simulink model "ABMS_FK_Optimization"  (R2024a)
settings: Solver=ode45  StartTime=0.0  StopTime=t1(end)  MaxStep=1e-4  RelTol=1e-3
model workspace (MAT data in the model file):
  SDO_OutputTimes = 0
values from neighbouring files (symbols this model uses):
  c_floor = 62.8188429312    [ForwardKinematicsReadyOptimization.mat]
  cAnkle = 1000    [ForwardKinematicsReadyOptimization.mat]
  cHat = 1000    [ForwardKinematicsReadyOptimization.mat]
  cHip = 1000    [ForwardKinematicsReadyOptimization.mat]
  cKnee = 1000    [ForwardKinematicsReadyOptimization.mat]
  d = 0.005    [ForwardKinematicsReadyOptimization.mat]
  dt = 0.00194789579158    [ForwardKinematicsReadyOptimization.mat]
  footCoG_x = 0.048032    [ForwardKinematicsReadyOptimization.mat]
  footCoG_y = 0.03081    [ForwardKinematicsReadyOptimization.mat]
  footHeight = 0.06162    [ForwardKinematicsReadyOptimization.mat]
  footInertia = 0.00070433888961    [ForwardKinematicsReadyOptimization.mat]
  footLength = 0.24016    [ForwardKinematicsReadyOptimization.mat]
  footMass = 0.82215    [ForwardKinematicsReadyOptimization.mat]
  hatCoG = -0.05733504    [ForwardKinematicsReadyOptimization.mat]
  hatInertia = 1.9582821044    [ForwardKinematicsReadyOptimization.mat]
  k_floor = 2646.94405241    [ForwardKinematicsReadyOptimization.mat]
  kAnkle = 11643.6295541    [ForwardKinematicsReadyOptimization.mat]
  kHat = 20655.7189422    [ForwardKinematicsReadyOptimization.mat]
  kHip = 10850.9172876    [ForwardKinematicsReadyOptimization.mat]
  kKnee = 36599.3663246    [ForwardKinematicsReadyOptimization.mat]
  L = 1.58    [ForwardKinematicsReadyOptimization.mat]
  M = 56.7    [ForwardKinematicsReadyOptimization.mat]
  omega_ankle_L = [-1.72946807619 -1.75737353503 -1.78034856033 -1.79855294145 -1.81216431593 -1.82137637434 -1.82639701034 -1.82744643093 -1.82475524177 -1.81856252257 -1.80911390714 -1.79665968238 ... (500 elements, 500x1)]    [ForwardKinematicsReadyOptimization.mat]
  omega_ankle_R = [2.03625246317 1.87895799946 1.71908308042 1.55696000935 1.39292869416 1.22733586468 1.06053424947 0.892881711684 0.724740343936 0.556475522401 0.388454920876 0.221047485982 ... (500 elements, 500x1)]    [ForwardKinematicsReadyOptimization.mat]
  omega_hip_L = [-0.280611688679 -0.311570063188 -0.345107260568 -0.38110500203 -0.419429739456 -0.459933358207 -0.502453986364 -0.546816904373 -0.592835548257 -0.640312598834 -0.68904114874 -0.738805938443 ... (500 elements, 500x1)]    [ForwardKinematicsReadyOptimization.mat]
  omega_hip_R = [2.436874577 2.50137810017 2.56518693791 2.62820305906 2.690326825 2.7514571145 2.81149146904 2.87032625968 2.92785687598 2.98397793742 3.03858352766 3.09156745152 ... (500 elements, 500x1)]    [ForwardKinematicsReadyOptimization.mat]
  omega_knee_L = [1.96123814792 1.91418307718 1.85419760709 1.78297919547 1.70210911406 1.61305682274 1.51718435711 1.41575071667 1.30991624212 1.20074697044 1.08921895698 0.976222554764 ... (500 elements, 500x1)]    [ForwardKinematicsReadyOptimization.mat]
  omega_knee_R = [-6.31491022355 -6.2996719536 -6.27749939257 -6.24831489493 -6.21206519479 -6.168721658 -6.11828036625 -6.06076203398 -5.99621176048 -5.92469862101 -5.84631510196 -5.76117638659 ... (500 elements, 500x1)]    [ForwardKinematicsReadyOptimization.mat]
  shankCoG = 0.02604156    [ForwardKinematicsReadyOptimization.mat]
  shankInertia = 0.0363273974795    [ForwardKinematicsReadyOptimization.mat]
  shankLength = 0.38868    [ForwardKinematicsReadyOptimization.mat]
  shankMass = 2.63655    [ForwardKinematicsReadyOptimization.mat]
  theta_ankle_L = [0.104089190059 0.10089407725 0.0976495615316 0.094363371469 0.0910429873004 0.0876956182925 0.0843281827148 0.0809472904543 0.0775592282756 0.0741699477128 0.070785055563 0.0674098069326 ... (500 elements, 500x1)]    [ForwardKinematicsReadyOptimization.mat]
  theta_ankle_R = [0.268664443161 0.271247145186 0.273677847781 0.275939163558 0.27801459569 0.279888613303 0.281546720628 0.282975519613 0.284162765692 0.28509741648 0.285769673205 0.286171014728 ... (500 elements, 500x1)]    [ForwardKinematicsReadyOptimization.mat]
  theta_hip_L = [0.203866490768 0.203326556251 0.202708469588 0.202008986109 0.201225063456 0.20035388195 0.199392863962 0.198339692183 0.197192326665 0.195949020524 0.194608334197 0.19316914817 ... (500 elements, 500x1)]    [ForwardKinematicsReadyOptimization.mat]
  theta_hip_R = [-0.0372016659367 -0.0333395086271 -0.0292594880672 -0.0249651189751 -0.0204604325022 -0.0157499604189 -0.0108387175733 -0.00573218271268 -0.000436277763004 0.00504265433304 0.010697873109 0.0165222652855 ... (500 elements, 500x1)]    [ForwardKinematicsReadyOptimization.mat]
  theta_knee_L = [-0.239993153363 -0.245883098322 -0.251093519717 -0.255698925452 -0.259765380933 -0.263351270801 -0.266508012215 -0.269280721542 -0.271708836309 -0.273826694261 -0.275664071344 -0.277246680395 ... (500 elements, 500x1)]    [ForwardKinematicsReadyOptimization.mat]
  theta_knee_R = [-0.820430486691 -0.832341256015 -0.844266598336 -0.856189608949 -0.868093439005 -0.879961330014 -0.891776648203 -0.903522918602 -0.915183858758 -0.926743411958 -0.938185779838 -0.949495454282 ... (500 elements, 500x1)]    [ForwardKinematicsReadyOptimization.mat]
  thighCoG = 0.0259357    [ForwardKinematicsReadyOptimization.mat]
  thighInertia = 0.0886409590374    [ForwardKinematicsReadyOptimization.mat]
  thighLength = 0.3871    [ForwardKinematicsReadyOptimization.mat]
  thighMass = 5.67    [ForwardKinematicsReadyOptimization.mat]
  x_hip = [-8.44173174878e-05 0.00319684354612 0.00644879199438 0.00967154739147 0.0128652983927 0.0160302986852 0.0191668628036 0.0222753620261 0.0253562203613 0.0284099106285 0.0314369506394 0.0344378994863 ... (500 elements, 500x1)]    [ForwardKinematicsReadyOptimization.mat]
  y_hip = [0.786844713626 0.786912596344 0.786989490296 0.787076184105 0.787173456036 0.787282069444 0.787402768296 0.787536272813 0.787683275238 0.787844435773 0.788020378698 0.788211688702 ... (500 elements, 500x1)]    [ForwardKinematicsReadyOptimization.mat]
undefined symbols (not defined in the file or in its folder): omega_hat, X, Y, y_heel, Z
libraries: nesl_utility x77, sm_lib x60
(part 2 of 3)

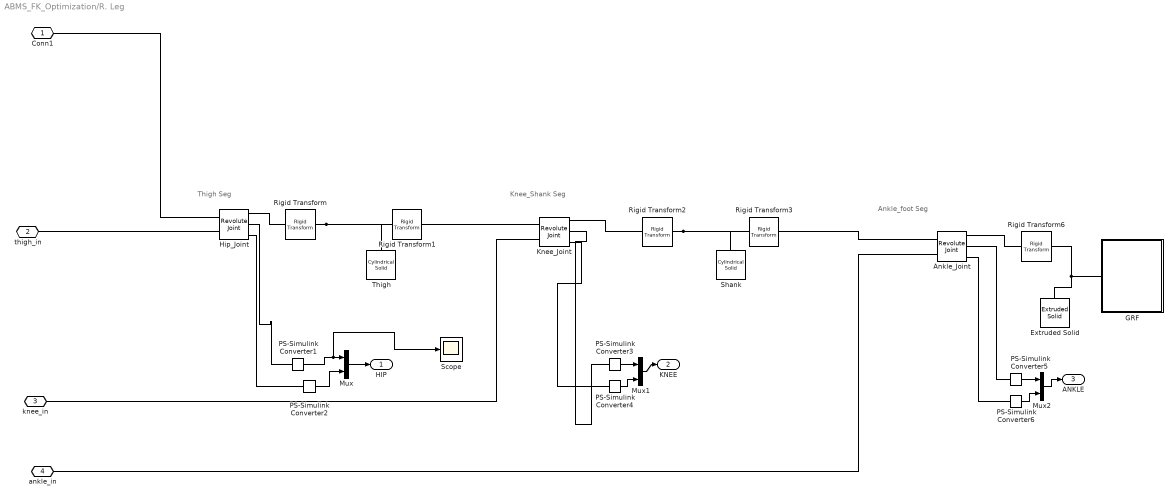
== system ABMS_FK_Optimization/R. Leg ==
  note: Ankle_foot Seg
  note: Knee_Shank Seg
  note: Thigh Seg
  Ankle_Joint : sm_lib/Joints/Revolute Joint  JointMode=Normal  CompositeWrenchDir=FollowerOnBase  CompositeWrenchFrame=BaseFrame  SenseConstraintForce=off  SenseConstraintTorque=off  SenseTotalForce=off  SenseTotalTorque=off  PositionTargetSpecify=on  PositionTargetPriority=High  PositionTargetValue=theta_ankle_R(1)  PositionTargetValueUnits=rad  VelocityTargetSpecify=on  VelocityTargetPriority=High  VelocityTargetValue=omega_ankle_R(1)  VelocityTargetValueUnits=rad/s  EquilibriumPosition=0  EquilibriumPositionUnits=deg  SpringStiffness=0  SpringStiffnessUnits=N*m/deg  DampingCoefficient=0  DampingCoefficientUnits=N*m/(deg/s)  LowerLimitSpecify=off  LowerLimitBound=-90  LowerLimitBoundUnits=deg  LowerLimitStiffness=1e4  LowerLimitStiffnessUnits=N*m/deg  LowerLimitDamping=10  LowerLimitDampingUnits=N*m/(deg/s)  LowerLimitTransitionRegionWidth=0.1  LowerLimitTransitionRegionWidthUnits=deg  UpperLimitSpecify=off  UpperLimitBound=90  UpperLimitBoundUnits=deg  UpperLimitStiffness=1e4  UpperLimitStiffnessUnits=N*m/deg  UpperLimitDamping=10  UpperLimitDampingUnits=N*m/(deg/s)  UpperLimitTransitionRegionWidth=0.1  UpperLimitTransitionRegionWidthUnits=deg  TorqueActuationMode=InputTorque  MotionActuationMode=ComputedMotion  SensePosition=on  SenseVelocity=on  SenseAcceleration=off  SenseTorqueForce=off  SenseLowerLimitTorqueForce=off  SenseUpperLimitTorqueForce=off
  Extruded Solid : sm_lib/Body Elements/Extruded Solid  ExtrusionType=General  PolygonNumSides=3  PolygonOuterRadius=footLength  PolygonOuterRadiusUnits=m  ExportEntireGeometry=off  ExtrusionCrossSection=[0 0; footLength 0; L*.0204 footHeight]  ExtrusionCrossSectionUnits=m  ExportConvexHullGeometry=off  ExtrusionLength=d  ExtrusionLengthUnits=m  InertiaType=Custom  BasedOnType=Mass  Density=1000  DensityUnits=kg/m^3  Mass=footMass  MassUnits=kg  CenterOfMass=[footCoG_x footCoG_y 0]  CenterOfMassUnits=m  MomentsOfInertia=[1 1 footInertia]  MomentsOfInertiaUnits=kg*m^2  ProductsOfInertia=[0 0 0]  ProductsOfInertiaUnits=kg*m^2  GraphicType=FromGeometry  MarkerShape=Sphere  MarkerSize=10  GraphicVisPropType=SimpleVisualProperties  GraphicDiffuseColor=[1.0 0.0 0.2]  GraphicOpacity=1.0  GraphicSpecularColor=[0.5 0.5 0.5 1.0]  GraphicAmbientColor=[0.15 0.15 0.15 1.0]  GraphicEmissiveColor=[0.0 0.0 0.0 1.0]  GraphicShininess=75  DoExposeReferenceFrame=on  SerializedFrames=<Frames><Frame><Id>Frame1</Id><Value><Name>CG</Name><Origin><Source>CenterOfMassFrame</Source><FeatureName></FeatureName></Origin><PrimaryAxis><DefinedDirection>+Z</DefinedDirection><Source>ReferenceFrame</Source><SourceDirection>+Z</SourceDirection><FeatureName></FeatureName></PrimaryAxis><SecondaryAxis><DefinedDirection>+X</DefinedDirection><Source>ReferenceFrame</Source><SourceDirection>+X</SourceDirection><FeatureName></FeatureName></SecondaryAxis></Value></Frame></Frames>
  GRF : Subsystem
  Hip_Joint : sm_lib/Joints/Revolute Joint  JointMode=Normal  CompositeWrenchDir=BaseOnFollower  CompositeWrenchFrame=BaseFrame  SenseConstraintForce=off  SenseConstraintTorque=off  SenseTotalForce=off  SenseTotalTorque=off  PositionTargetSpecify=on  PositionTargetPriority=High  PositionTargetValue=theta_hip_R(1)  PositionTargetValueUnits=rad  VelocityTargetSpecify=on  VelocityTargetPriority=High  VelocityTargetValue=omega_hip_R(1)  VelocityTargetValueUnits=rad/s  EquilibriumPosition=0  EquilibriumPositionUnits=deg  SpringStiffness=0  SpringStiffnessUnits=N*m/deg  DampingCoefficient=0  DampingCoefficientUnits=N*m/(deg/s)  LowerLimitSpecify=off  LowerLimitBound=-90  LowerLimitBoundUnits=deg  LowerLimitStiffness=1e4  LowerLimitStiffnessUnits=N*m/deg  LowerLimitDamping=10  LowerLimitDampingUnits=N*m/(deg/s)  LowerLimitTransitionRegionWidth=0.1  LowerLimitTransitionRegionWidthUnits=deg  UpperLimitSpecify=off  UpperLimitBound=90  UpperLimitBoundUnits=deg  UpperLimitStiffness=1e4  UpperLimitStiffnessUnits=N*m/deg  UpperLimitDamping=10  UpperLimitDampingUnits=N*m/(deg/s)  UpperLimitTransitionRegionWidth=0.1  UpperLimitTransitionRegionWidthUnits=deg  TorqueActuationMode=InputTorque  MotionActuationMode=ComputedMotion  SensePosition=on  SenseVelocity=on  SenseAcceleration=off  SenseTorqueForce=off  SenseLowerLimitTorqueForce=off  SenseUpperLimitTorqueForce=off
  Knee_Joint : sm_lib/Joints/Revolute Joint  JointMode=Normal  CompositeWrenchDir=FollowerOnBase  CompositeWrenchFrame=BaseFrame  SenseConstraintForce=off  SenseConstraintTorque=off  SenseTotalForce=off  SenseTotalTorque=off  PositionTargetSpecify=on  PositionTargetPriority=High  PositionTargetValue=theta_knee_R(1)  PositionTargetValueUnits=rad  VelocityTargetSpecify=on  VelocityTargetPriority=High  VelocityTargetValue=omega_knee_R(1)  VelocityTargetValueUnits=rad/s  EquilibriumPosition=0  EquilibriumPositionUnits=deg  SpringStiffness=0  SpringStiffnessUnits=N*m/deg  DampingCoefficient=0  DampingCoefficientUnits=N*m/(deg/s)  LowerLimitSpecify=off  LowerLimitBound=-90  LowerLimitBoundUnits=deg  LowerLimitStiffness=1e4  LowerLimitStiffnessUnits=N*m/deg  LowerLimitDamping=10  LowerLimitDampingUnits=N*m/(deg/s)  LowerLimitTransitionRegionWidth=0.1  LowerLimitTransitionRegionWidthUnits=deg  UpperLimitSpecify=off  UpperLimitBound=90  UpperLimitBoundUnits=deg  UpperLimitStiffness=1e4  UpperLimitStiffnessUnits=N*m/deg  UpperLimitDamping=10  UpperLimitDampingUnits=N*m/(deg/s)  UpperLimitTransitionRegionWidth=0.1  UpperLimitTransitionRegionWidthUnits=deg  TorqueActuationMode=InputTorque  MotionActuationMode=ComputedMotion  SensePosition=on  SenseVelocity=on  SenseAcceleration=off  SenseTorqueForce=off  SenseLowerLimitTorqueForce=off  SenseUpperLimitTorqueForce=off
  Mux : Mux  Inputs=2
  Mux1 : Mux  Inputs=2
  Mux2 : Mux  Inputs=2
  PS-Simulink Converter{1..6} (6 alike) : nesl_utility/PS-Simulink Converter  PhysicalDomain=network_engine_domain  SubClassName=ps_output  LeftPortType=input  RightPortType=output  PseudoPeriodic=off  Frequencies=[]  VectorFormat=1-D array  Unit=inherit  AffineConversion=off
  Rigid Transform : sm_lib/Frames and Transforms/Rigid Transform  RotationMethod=StandardAxis  FollAlignAxisA=+X  BaseAlignAxisA=+Y  FollAlignAxisB=+Y  BaseAlignAxisB=+Z  RotationStandardAxis=+X  RotationAngle=90  RotationAngleUnits=deg  RotationArbitraryAxis=[0 0 1]  RotationSequenceAxes=FollowerAxes  RotationSequence=XYX  RotationSequenceAngles=[0 0 0]  RotationSequenceAnglesUnits=deg  RotationMatrix=[1 0 0; 0 1 0; 0 0 1]  Quaternion=[1 0 0 0]  TranslationMethod=Cartesian  TranslationCartesianOffset=[0 0 thighLength/2]  TranslationCartesianOffsetUnits=m  TranslationStandardAxis=+Z  TranslationStandardOffset=thighLength/2  TranslationStandardOffsetUnits=m  TranslationROffset=0  TranslationROffsetUnits=m  TranslationThetaOffset=0  TranslationThetaOffsetUnits=deg  TranslationZOffset=0  TranslationZOffsetUnits=m
  Rigid Transform1 : sm_lib/Frames and Transforms/Rigid Transform  RotationMethod=StandardAxis  FollAlignAxisA=+X  BaseAlignAxisA=+Y  FollAlignAxisB=+Y  BaseAlignAxisB=+Z  RotationStandardAxis=+X  RotationAngle=90  RotationAngleUnits=deg  RotationArbitraryAxis=[0 0 1]  RotationSequenceAxes=FollowerAxes  RotationSequence=XYX  RotationSequenceAngles=[0 0 0]  RotationSequenceAnglesUnits=deg  RotationMatrix=[1 0 0; 0 1 0; 0 0 1]  Quaternion=[1 0 0 0]  TranslationMethod=StandardAxis  TranslationCartesianOffset=[0 0 0]  TranslationCartesianOffsetUnits=m  TranslationStandardAxis=-Z  TranslationStandardOffset=thighLength/2  TranslationStandardOffsetUnits=m  TranslationROffset=0  TranslationROffsetUnits=m  TranslationThetaOffset=0  TranslationThetaOffsetUnits=deg  TranslationZOffset=0  TranslationZOffsetUnits=m
  Rigid Transform2 : sm_lib/Frames and Transforms/Rigid Transform  RotationMethod=StandardAxis  FollAlignAxisA=+X  BaseAlignAxisA=+Y  FollAlignAxisB=+Y  BaseAlignAxisB=+Z  RotationStandardAxis=+X  RotationAngle=90  RotationAngleUnits=deg  RotationArbitraryAxis=[0 0 1]  RotationSequenceAxes=FollowerAxes  RotationSequence=XYX  RotationSequenceAngles=[0 0 0]  RotationSequenceAnglesUnits=deg  RotationMatrix=[1 0 0; 0 1 0; 0 0 1]  Quaternion=[1 0 0 0]  TranslationMethod=StandardAxis  TranslationCartesianOffset=[0 0 0]  TranslationCartesianOffsetUnits=m  TranslationStandardAxis=+Z  TranslationStandardOffset=shankLength/2  TranslationStandardOffsetUnits=m  TranslationROffset=0  TranslationROffsetUnits=m  TranslationThetaOffset=0  TranslationThetaOffsetUnits=deg  TranslationZOffset=0  TranslationZOffsetUnits=m
  Rigid Transform3 : sm_lib/Frames and Transforms/Rigid Transform  RotationMethod=StandardAxis  FollAlignAxisA=+X  BaseAlignAxisA=+Y  FollAlignAxisB=+Y  BaseAlignAxisB=+Z  RotationStandardAxis=+X  RotationAngle=90  RotationAngleUnits=deg  RotationArbitraryAxis=[0 0 1]  RotationSequenceAxes=FollowerAxes  RotationSequence=XYX  RotationSequenceAngles=[0 0 0]  RotationSequenceAnglesUnits=deg  RotationMatrix=[1 0 0; 0 1 0; 0 0 1]  Quaternion=[1 0 0 0]  TranslationMethod=StandardAxis  TranslationCartesianOffset=[0 0 0]  TranslationCartesianOffsetUnits=m  TranslationStandardAxis=-Z  TranslationStandardOffset=shankLength/2  TranslationStandardOffsetUnits=m  TranslationROffset=0  TranslationROffsetUnits=m  TranslationThetaOffset=0  TranslationThetaOffsetUnits=deg  TranslationZOffset=0  TranslationZOffsetUnits=m
  Rigid Transform6 : sm_lib/Frames and Transforms/Rigid Transform  RotationMethod=None  FollAlignAxisA=+X  BaseAlignAxisA=+Y  FollAlignAxisB=+Y  BaseAlignAxisB=+Z  RotationStandardAxis=+Z  RotationAngle=0.0  RotationAngleUnits=deg  RotationArbitraryAxis=[0 0 1]  RotationSequenceAxes=FollowerAxes  RotationSequence=XYX  RotationSequenceAngles=[0 0 0]  RotationSequenceAnglesUnits=deg  RotationMatrix=[1 0 0; 0 1 0; 0 0 1]  Quaternion=[1 0 0 0]  TranslationMethod=Cartesian  TranslationCartesianOffset=[0.0204*L 0.039*L 0]  TranslationCartesianOffsetUnits=m  TranslationStandardAxis=+Z  TranslationStandardOffset=0  TranslationStandardOffsetUnits=m  TranslationROffset=0  TranslationROffsetUnits=m  TranslationThetaOffset=0  TranslationThetaOffsetUnits=deg  TranslationZOffset=0  TranslationZOffsetUnits=m
  Scope : Scope
  Shank : sm_lib/Body Elements/Cylindrical Solid  CylinderRadius=d/2  CylinderRadiusUnits=m  CylinderLength=shankLength  CylinderLengthUnits=m  ExportEntireGeometry=off  InertiaType=Custom  BasedOnType=Mass  Density=1000  DensityUnits=kg/m^3  Mass=shankMass  MassUnits=kg  CenterOfMass=[0 0 shankCoG]  CenterOfMassUnits=m  MomentsOfInertia=[shankInertia shankInertia 0]  MomentsOfInertiaUnits=kg*m^2  ProductsOfInertia=[0 0 0]  ProductsOfInertiaUnits=kg*m^2  GraphicType=FromGeometry  MarkerShape=Sphere  MarkerSize=10  GraphicVisPropType=SimpleVisualProperties  GraphicDiffuseColor=[0.0 0.2 1.0]  GraphicOpacity=1.0  GraphicSpecularColor=[0.5 0.5 0.5 1.0]  GraphicAmbientColor=[0.15 0.15 0.15 1.0]  GraphicEmissiveColor=[0.0 0.0 0.0 1.0]  GraphicShininess=75  DoExposeReferenceFrame=on  SerializedFrames=<Frames><Frame><Id>Frame1</Id><Value><Name>CG</Name><Origin><Source>CenterOfMassFrame</Source><FeatureName></FeatureName></Origin><PrimaryAxis><DefinedDirection>+Z</DefinedDirection><Source>ReferenceFrame</Source><SourceDirection>+Z</SourceDirection><FeatureName></FeatureName></PrimaryAxis><SecondaryAxis><DefinedDirection>+X</DefinedDirection><Source>ReferenceFrame</Source><SourceDirection>+X</SourceDirection><FeatureName></FeatureName></SecondaryAxis></Value></Frame></Frames>
  Thigh : sm_lib/Body Elements/Cylindrical Solid  CylinderRadius=d/2  CylinderRadiusUnits=m  CylinderLength=thighLength  CylinderLengthUnits=m  ExportEntireGeometry=off  InertiaType=Custom  BasedOnType=Mass  Density=1000  DensityUnits=kg/m^3  Mass=thighMass  MassUnits=kg  CenterOfMass=[0 0 thighCoG]  CenterOfMassUnits=m  MomentsOfInertia=[thighInertia thighInertia 0]  MomentsOfInertiaUnits=kg*m^2  ProductsOfInertia=[0 0 0]  ProductsOfInertiaUnits=kg*m^2  GraphicType=FromGeometry  MarkerShape=Sphere  MarkerSize=10  GraphicVisPropType=SimpleVisualProperties  GraphicDiffuseColor=[0.0 0.0 0.0]  GraphicOpacity=1.0  GraphicSpecularColor=[0.5 0.5 0.5 1.0]  GraphicAmbientColor=[0.15 0.15 0.15 1.0]  GraphicEmissiveColor=[0.0 0.0 0.0 1.0]  GraphicShininess=75  DoExposeReferenceFrame=on  SerializedFrames=<Frames><Frame><Id>Frame1</Id><Value><Name>CG</Name><Origin><Source>CenterOfMassFrame</Source><FeatureName></FeatureName></Origin><PrimaryAxis><DefinedDirection>+Z</DefinedDirection><Source>ReferenceFrame</Source><SourceDirection>+Z</SourceDirection><FeatureName></FeatureName></PrimaryAxis><SecondaryAxis><DefinedDirection>+X</DefinedDirection><Source>ReferenceFrame</Source><SourceDirection>+X</SourceDirection><FeatureName></FeatureName></SecondaryAxis></Value></Frame></Frames>
  Conn1 : PMIOPort  Side=Left
  thigh_in : PMIOPort  Port=2  Side=Left
  knee_in : PMIOPort  Port=3  Side=Left
  ankle_in : PMIOPort  Port=4  Side=Left
  HIP : Outport
  KNEE : Outport  Port=2
  ANKLE : Outport  Port=3
  wires:
  PS-Simulink Converter2/1 -> Mux/2
  PS-Simulink Converter4/1 -> Mux1/2
  PS-Simulink Converter1/1 -> Scope/1, Mux/1
  Mux/1 -> HIP/1
  PS-Simulink Converter3/1 -> Mux1/1
  Mux1/1 -> KNEE/1
  PS-Simulink Converter5/1 -> Mux2/1
  Mux2/1 -> ANKLE/1
  PS-Simulink Converter6/1 -> Mux2/2
  connections:
  Rigid Transform/LConn1 -- Rigid Transform1/LConn1 -- Thigh/RConn1
  Knee_Joint/LConn1 -- Rigid Transform1/RConn1
  Hip_Joint/RConn1 -- Rigid Transform/RConn1
  Rigid Transform2/LConn1 -- Shank/RConn1 -- Rigid Transform3/LConn1
  Rigid Transform6/RConn1 -- Ankle_Joint/RConn1
  Rigid Transform2/RConn1 -- Knee_Joint/RConn1
  Rigid Transform3/RConn1 -- Ankle_Joint/LConn1
  Hip_Joint/LConn1 -- Conn1/RConn1
  PS-Simulink Converter1/LConn1 -- Hip_Joint/RConn2
  Extruded Solid/RConn1 -- GRF/LConn1 -- Rigid Transform6/LConn1
  PS-Simulink Converter4/LConn1 -- Knee_Joint/RConn3
  PS-Simulink Converter3/LConn1 -- Knee_Joint/RConn2
  PS-Simulink Converter2/LConn1 -- Hip_Joint/RConn3
  Ankle_Joint/RConn2 -- PS-Simulink Converter5/LConn1
  PS-Simulink Converter6/LConn1 -- Ankle_Joint/RConn3
  thigh_in/RConn1 -- Hip_Joint/LConn2
  knee_in/RConn1 -- Knee_Joint/LConn2
  ankle_in/RConn1 -- Ankle_Joint/LConn2

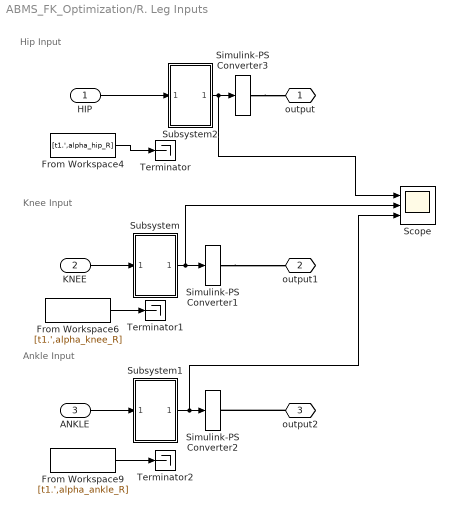
== system ABMS_FK_Optimization/R. Leg Inputs ==
  note: Ankle Input
  note: Knee Input
  note: Hip Input
  HIP : Inport
  KNEE : Inport  Port=2
  ANKLE : Inport  Port=3
  From Workspace4 : FromWorkspace  VariableName=[t1.',alpha_hip_R]  SampleTime=dt
  From Workspace6 : FromWorkspace  VariableName=[t1.',alpha_knee_R]  SampleTime=dt
  From Workspace9 : FromWorkspace  VariableName=[t1.',alpha_ankle_R]  SampleTime=dt
  Scope : Scope  NumInputPorts=3
  Simulink-PS Converter1 : nesl_utility/Simulink-PS Converter  PhysicalDomain=network_engine_domain  SubClassName=ps_input  LeftPortType=input  RightPortType=output  PseudoPeriodic=off  Frequencies=[]  NoiseDistribution=none  NoiseParameters=[]  Unit=1  AffineConversion=off  FilteringAndDerivatives=provide  SimscapeFilterOrder=2  InputFilterTimeConstant=0.001  UdotUserProvided=0
  Simulink-PS Converter2 : nesl_utility/Simulink-PS Converter  PhysicalDomain=network_engine_domain  SubClassName=ps_input  LeftPortType=input  RightPortType=output  PseudoPeriodic=off  Frequencies=[]  NoiseDistribution=none  NoiseParameters=[]  Unit=1  AffineConversion=off  FilteringAndDerivatives=provide  SimscapeFilterOrder=2  InputFilterTimeConstant=0.001  UdotUserProvided=0
  Simulink-PS Converter3 : nesl_utility/Simulink-PS Converter  PhysicalDomain=network_engine_domain  SubClassName=ps_input  LeftPortType=input  RightPortType=output  PseudoPeriodic=off  Frequencies=[]  NoiseDistribution=none  NoiseParameters=[]  Unit=1  AffineConversion=off  FilteringAndDerivatives=provide  SimscapeFilterOrder=2  InputFilterTimeConstant=0.001  UdotUserProvided=0
  Subsystem : Subsystem
  Subsystem1 : Subsystem
  Subsystem2 : Subsystem
  Terminator : Terminator
  Terminator1 : Terminator
  Terminator2 : Terminator
  output : PMIOPort  Side=Right
  output1 : PMIOPort  Port=2  Side=Right
  output2 : PMIOPort  Port=3  Side=Right
  wires:
  KNEE/1 -> Subsystem/1(In1)
  Subsystem/1(Out1) -> Scope/2, Simulink-PS Converter1/1
  ANKLE/1 -> Subsystem1/1(In1)
  Subsystem1/1(Out1) -> Scope/3, Simulink-PS Converter2/1
  HIP/1 -> Subsystem2/1(1)
  Subsystem2/1(Out1) -> Scope/1, Simulink-PS Converter3/1
  From Workspace4/1 -> Terminator/1
  From Workspace6/1 -> Terminator1/1
  From Workspace9/1 -> Terminator2/1
  connections:
  output2/RConn1 -- Simulink-PS Converter2/RConn1
  Simulink-PS Converter1/RConn1 -- output1/RConn1
  Simulink-PS Converter3/RConn1 -- output/RConn1

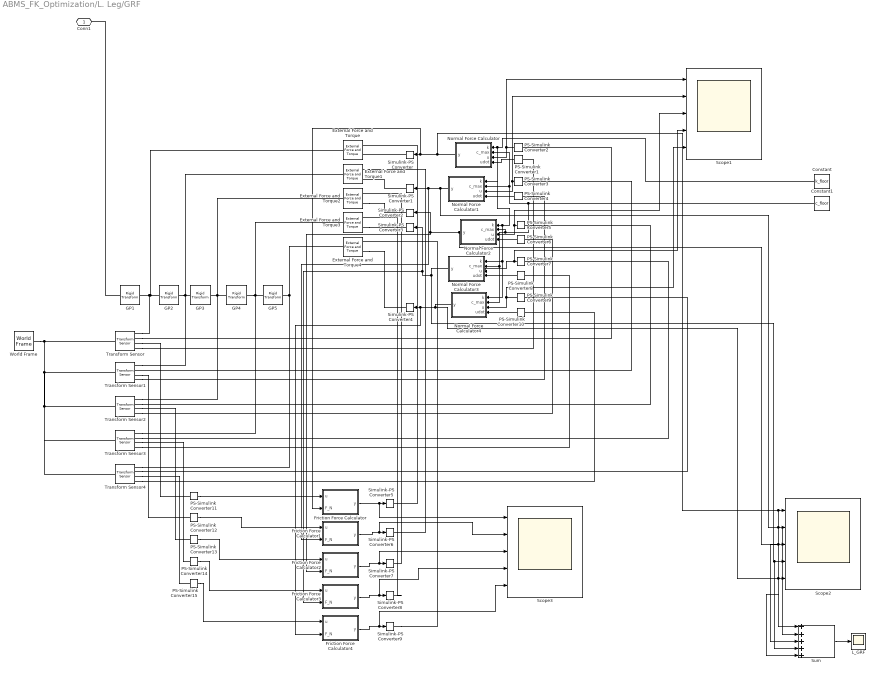
== system ABMS_FK_Optimization/L. Leg/GRF ==
  Constant : Constant  Value=k_floor
  Constant1 : Constant  Value=c_floor
  External Force and Torque{,1..4} (5 alike) : sm_lib/Forces and Torques/External Force and Torque  EnableForceX=on  EnableForceY=on  EnableForceZ=off  EnableForce=off  ForceResolutionFrame=World  EnableTorqueX=off  EnableTorqueY=off  EnableTorqueZ=off  EnableTorque=off  TorqueResolutionFrame=AttachedFrame
  Friction Force Calculator : MATLAB Function  TreatAsAtomicUnit=on
  Friction Force Calculator1 : MATLAB Function  TreatAsAtomicUnit=on
  Friction Force Calculator2 : MATLAB Function  TreatAsAtomicUnit=on
  Friction Force Calculator3 : MATLAB Function  TreatAsAtomicUnit=on
  Friction Force Calculator4 : MATLAB Function  TreatAsAtomicUnit=on
  GP1 : sm_lib/Frames and Transforms/Rigid Transform  RotationMethod=None  FollAlignAxisA=+X  BaseAlignAxisA=+Y  FollAlignAxisB=+Y  BaseAlignAxisB=+Z  RotationStandardAxis=+Z  RotationAngle=0.0  RotationAngleUnits=deg  RotationArbitraryAxis=[0 0 1]  RotationSequenceAxes=FollowerAxes  RotationSequence=XYX  RotationSequenceAngles=[0 0 0]  RotationSequenceAnglesUnits=deg  RotationMatrix=[1 0 0; 0 1 0; 0 0 1]  Quaternion=[1 0 0 0]  TranslationMethod=None  TranslationCartesianOffset=[0 0 0]  TranslationCartesianOffsetUnits=m  TranslationStandardAxis=-X  TranslationStandardOffset=d/2  TranslationStandardOffsetUnits=m  TranslationROffset=0  TranslationROffsetUnits=m  TranslationThetaOffset=0  TranslationThetaOffsetUnits=deg  TranslationZOffset=0  TranslationZOffsetUnits=m
  GP{2..5} (4 alike) : sm_lib/Frames and Transforms/Rigid Transform  RotationMethod=None  FollAlignAxisA=+X  BaseAlignAxisA=+Y  FollAlignAxisB=+Y  BaseAlignAxisB=+Z  RotationStandardAxis=+Z  RotationAngle=0.0  RotationAngleUnits=deg  RotationArbitraryAxis=[0 0 1]  RotationSequenceAxes=FollowerAxes  RotationSequence=XYX  RotationSequenceAngles=[0 0 0]  RotationSequenceAnglesUnits=deg  RotationMatrix=[1 0 0; 0 1 0; 0 0 1]  Quaternion=[1 0 0 0]  TranslationMethod=StandardAxis  TranslationCartesianOffset=[0 0 0]  TranslationCartesianOffsetUnits=m  TranslationStandardAxis=+X  TranslationStandardOffset=footLength/4  TranslationStandardOffsetUnits=m  TranslationROffset=0  TranslationROffsetUnits=m  TranslationThetaOffset=0  TranslationThetaOffsetUnits=deg  TranslationZOffset=0  TranslationZOffsetUnits=m
  L_GRF : Scope
  Normal Force Calculator : MATLAB Function  TreatAsAtomicUnit=on
  Normal Force Calculator1 : MATLAB Function  TreatAsAtomicUnit=on
  Normal Force Calculator2 : MATLAB Function  TreatAsAtomicUnit=on
  Normal Force Calculator3 : MATLAB Function  TreatAsAtomicUnit=on
  Normal Force Calculator4 : MATLAB Function  TreatAsAtomicUnit=on
  PS-Simulink Converter{1..15} (15 alike) : nesl_utility/PS-Simulink Converter  PhysicalDomain=network_engine_domain  SubClassName=ps_output  LeftPortType=input  RightPortType=output  PseudoPeriodic=off  Frequencies=[]  VectorFormat=1-D array  Unit=inherit  AffineConversion=off
  Scope1 : Scope  NumInputPorts=5
  Scope2 : Scope  NumInputPorts=5
  Scope3 : Scope  NumInputPorts=5
  Simulink-PS Converter{,1..9} (10 alike) : nesl_utility/Simulink-PS Converter  PhysicalDomain=network_engine_domain  SubClassName=ps_input  LeftPortType=input  RightPortType=output  PseudoPeriodic=off  Frequencies=[]  NoiseDistribution=none  NoiseParameters=[]  Unit=1  AffineConversion=off  FilteringAndDerivatives=provide  SimscapeFilterOrder=1  InputFilterTimeConstant=0.001  UdotUserProvided=0
  Sum : Sum  Inputs=+++++
  Transform Sensor{,1..4} (5 alike) : sm_lib/Frames and Transforms/Transform Sensor  MeasurementFrame=World  RotationSequence=XYX  SenseAngle=off  SenseAxis=off  SenseQ=off  SenseR=off  SenseRotationSequence=off  SenseOmegaX=off  SenseOmegaY=off  SenseOmegaZ=off  SenseOmega=off  SenseQDot=off  SenseRDot=off  SenseRotationSequenceDot=off  SenseAlphaX=off  SenseAlphaY=off  SenseAlphaZ=off  SenseAlpha=off  SenseQDDot=off  SenseRDDot=off  SenseX=off  SenseY=on  SenseZ=off  SenseXYZ=off  SenseRad=off  SenseAzim=off  SenseDist=off  SenseInc=off  SenseXDot=on  SenseYDot=on  SenseZDot=off  SenseXYZDot=off  SenseRadDot=off  SenseAzimDot=off  SenseDistDot=off  SenseIncDot=off  SenseXDDot=off  SenseYDDot=off  SenseZDDot=off  SenseXYZDDot=off  SenseRadDDot=off  SenseAzimDDot=off  SenseDistDDot=off  SenseIncDDot=off
  World Frame : sm_lib/Frames and Transforms/World Frame
  Conn1 : PMIOPort  Side=Left
  wires:
  PS-Simulink Converter2/1 -> Scope1/1, Normal Force Calculator/3(u)
  Normal Force Calculator4/1(y) -> Sum/5, Scope2/5, Friction Force Calculator4/2(F_N), Simulink-PS Converter4/1
  Friction Force Calculator3/1(y) -> Scope3/4, Simulink-PS Converter8/1
  Normal Force Calculator/1(y) -> Sum/1, Scope2/1, Friction Force Calculator/2(F_N), Simulink-PS Converter/1
  PS-Simulink Converter9/1 -> Normal Force Calculator4/3(u), Scope1/5
  Friction Force Calculator4/1(y) -> Scope3/5, Simulink-PS Converter9/1
  PS-Simulink Converter5/1 -> Normal Force Calculator2/3(u), Scope1/3
  PS-Simulink Converter15/1 -> Friction Force Calculator4/1(u)
  PS-Simulink Converter10/1 -> Normal Force Calculator4/4(udot)
  PS-Simulink Converter8/1 -> Normal Force Calculator3/4(udot)
  PS-Simulink Converter12/1 -> Friction Force Calculator1/1(u)
  Normal Force Calculator1/1(y) -> Sum/2, Scope2/2, Friction Force Calculator1/2(F_N), Simulink-PS Converter1/1
  PS-Simulink Converter13/1 -> Friction Force Calculator2/1(u)
  PS-Simulink Converter3/1 -> Normal Force Calculator1/3(u), Scope1/2
  PS-Simulink Converter4/1 -> Normal Force Calculator1/4(udot)
  Friction Force Calculator2/1(y) -> Scope3/3, Simulink-PS Converter7/1
  PS-Simulink Converter1/1 -> Normal Force Calculator/4(udot)
  Friction Force Calculator/1(y) -> Scope3/1, Simulink-PS Converter5/1
  Normal Force Calculator3/1(y) -> Scope2/4, Sum/4, Friction Force Calculator3/2(F_N), Simulink-PS Converter3/1
  PS-Simulink Converter7/1 -> Normal Force Calculator3/3(u), Scope1/4
  Constant1/1 -> Normal Force Calculator4/2(c_max), Normal Force Calculator3/2(c_max), Normal Force Calculator2/2(c_max), Normal Force Calculator1/2(c_max), Normal Force Calculator/2(c_max)
  PS-Simulink Converter6/1 -> Normal Force Calculator2/4(udot)
  Normal Force Calculator2/1(y) -> Sum/3, Scope2/3, Friction Force Calculator2/2(F_N), Simulink-PS Converter2/1
  Friction Force Calculator1/1(y) -> Scope3/2, Simulink-PS Converter6/1
  Sum/1 -> L_GRF/1
  Constant/1 -> Normal Force Calculator3/1(k), Normal Force Calculator4/1(k), Normal Force Calculator2/1(k), Normal Force Calculator1/1(k), Normal Force Calculator/1(k)
  PS-Simulink Converter14/1 -> Friction Force Calculator3/1(u)
  PS-Simulink Converter11/1 -> Friction Force Calculator/1(u)
  connections:
  Simulink-PS Converter5/RConn1 -- External Force and Torque/LConn1
  External Force and Torque2/LConn2 -- Simulink-PS Converter2/RConn1
  GP3/RConn1 -- External Force and Torque2/RConn1 -- Transform Sensor2/RConn1 -- GP4/LConn1
  GP2/LConn1 -- External Force and Torque/RConn1 -- Transform Sensor/RConn1 -- GP1/RConn1
  Transform Sensor2/RConn4 -- PS-Simulink Converter6/LConn1
  World Frame/RConn1 -- Transform Sensor4/LConn1 -- Transform Sensor3/LConn1 -- Transform Sensor2/LConn1 -- Transform Sensor1/LConn1 -- Transform Sensor/LConn1
  Transform Sensor3/RConn4 -- PS-Simulink Converter8/LConn1
  External Force and Torque1/LConn1 -- Simulink-PS Converter6/RConn1
  Transform Sensor3/RConn3 -- PS-Simulink Converter14/LConn1
  Transform Sensor4/RConn1 -- External Force and Torque4/RConn1 -- GP5/RConn1
  External Force and Torque3/LConn2 -- Simulink-PS Converter3/RConn1
  GP4/RConn1 -- External Force and Torque3/RConn1 -- Transform Sensor3/RConn1 -- GP5/LConn1
  Transform Sensor/RConn2 -- PS-Simulink Converter2/LConn1
  Transform Sensor2/RConn3 -- PS-Simulink Converter13/LConn1
  GP3/LConn1 -- External Force and Torque1/RConn1 -- Transform Sensor1/RConn1 -- GP2/RConn1
  Simulink-PS Converter7/RConn1 -- External Force and Torque2/LConn1
  Simulink-PS Converter8/RConn1 -- External Force and Torque3/LConn1
  PS-Simulink Converter3/LConn1 -- Transform Sensor1/RConn2
  Simulink-PS Converter1/RConn1 -- External Force and Torque1/LConn2
  Transform Sensor/RConn4 -- PS-Simulink Converter1/LConn1
  Transform Sensor4/RConn4 -- PS-Simulink Converter10/LConn1
  Transform Sensor4/RConn2 -- PS-Simulink Converter9/LConn1
  Transform Sensor/RConn3 -- PS-Simulink Converter11/LConn1
  Transform Sensor1/RConn4 -- PS-Simulink Converter4/LConn1
  Simulink-PS Converter/RConn1 -- External Force and Torque/LConn2
  Transform Sensor3/RConn2 -- PS-Simulink Converter7/LConn1
  Transform Sensor2/RConn2 -- PS-Simulink Converter5/LConn1
  Simulink-PS Converter9/RConn1 -- External Force and Torque4/LConn1
  Transform Sensor1/RConn3 -- PS-Simulink Converter12/LConn1
  Transform Sensor4/RConn3 -- PS-Simulink Converter15/LConn1
  External Force and Torque4/LConn2 -- Simulink-PS Converter4/RConn1
  GP1/LConn1 -- Conn1/RConn1

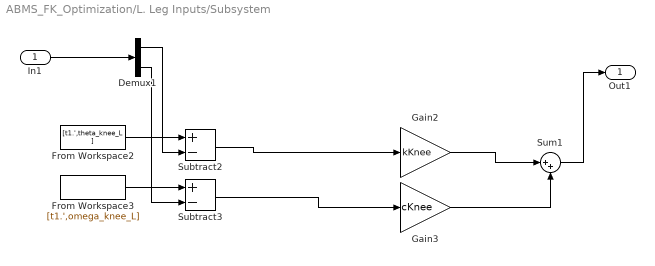
== system ABMS_FK_Optimization/L. Leg Inputs/Subsystem ==
  In1 : Inport
  Demux1 : Demux  Outputs=2
  From Workspace2 : FromWorkspace  VariableName=[t1.',theta_knee_L ]  SampleTime=dt
  From Workspace3 : FromWorkspace  VariableName=[t1.',omega_knee_L]  SampleTime=dt
  Gain2 : Gain  Gain=kKnee
  Gain3 : Gain  Gain=cKnee
  Subtract2 : Sum  Inputs=+-
  Subtract3 : Sum  Inputs=+-
  Sum1 : Sum  Inputs=|++
  Out1 : Outport
  wires:
  Subtract2/1 -> Gain2/1
  Gain3/1 -> Sum1/2
  Gain2/1 -> Sum1/1
  Demux1/1 -> Subtract2/2
  Demux1/2 -> Subtract3/2
  Subtract3/1 -> Gain3/1
  In1/1 -> Demux1/1
  Sum1/1 -> Out1/1
  From Workspace2/1 -> Subtract2/1
  From Workspace3/1 -> Subtract3/1

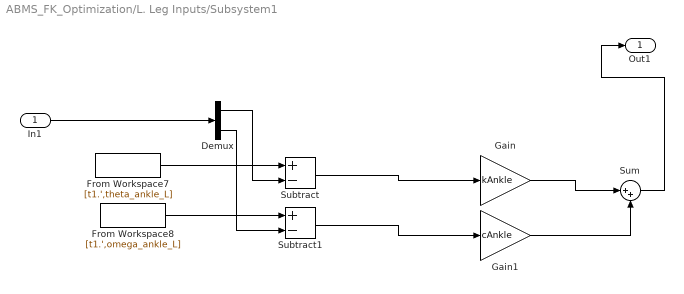
== system ABMS_FK_Optimization/L. Leg Inputs/Subsystem1 ==
  In1 : Inport
  Demux : Demux  Outputs=2
  From Workspace7 : FromWorkspace  VariableName=[t1.',theta_ankle_L]  SampleTime=dt
  From Workspace8 : FromWorkspace  VariableName=[t1.',omega_ankle_L]  SampleTime=dt
  Gain : Gain  Gain=kAnkle
  Gain1 : Gain  Gain=cAnkle
  Subtract : Sum  Inputs=+-
  Subtract1 : Sum  Inputs=+-
  Sum : Sum  Inputs=|++
  Out1 : Outport
  wires:
  From Workspace7/1 -> Subtract/1
  Subtract/1 -> Gain/1
  From Workspace8/1 -> Subtract1/1
  Demux/1 -> Subtract/2
  Demux/2 -> Subtract1/2
  Gain1/1 -> Sum/2
  Gain/1 -> Sum/1
  Subtract1/1 -> Gain1/1
  In1/1 -> Demux/1
  Sum/1 -> Out1/1

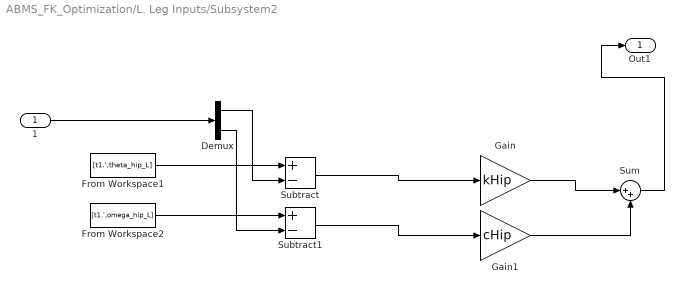
== system ABMS_FK_Optimization/L. Leg Inputs/Subsystem2 ==
  1 : Inport
  Demux : Demux  Outputs=2
  From Workspace1 : FromWorkspace  VariableName=[t1.',theta_hip_L]  SampleTime=dt
  From Workspace2 : FromWorkspace  VariableName=[t1.',omega_hip_L]  SampleTime=dt
  Gain : Gain  Gain=kHip
  Gain1 : Gain  Gain=cHip
  Subtract : Sum  Inputs=+-
  Subtract1 : Sum  Inputs=+-
  Sum : Sum  Inputs=|++
  Out1 : Outport
  wires:
  From Workspace1/1 -> Subtract/1
  Subtract/1 -> Gain/1
  From Workspace2/1 -> Subtract1/1
  Demux/1 -> Subtract/2
  Demux/2 -> Subtract1/2
  Gain1/1 -> Sum/2
  Gain/1 -> Sum/1
  Subtract1/1 -> Gain1/1
  1/1 -> Demux/1
  Sum/1 -> Out1/1

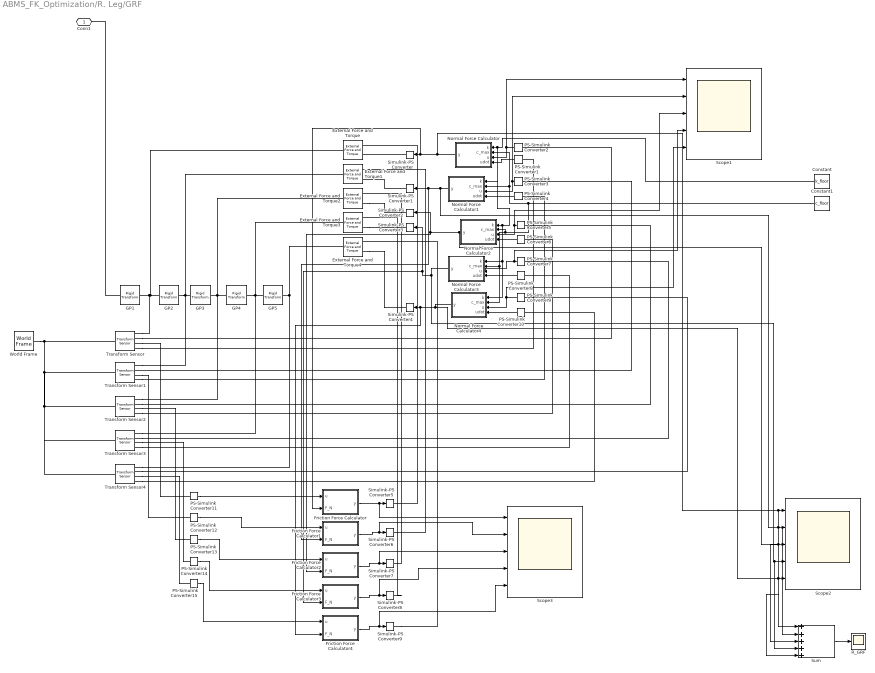
== system ABMS_FK_Optimization/R. Leg/GRF ==
  Constant : Constant  Value=k_floor
  Constant1 : Constant  Value=c_floor
  External Force and Torque{,1..4} (5 alike) : sm_lib/Forces and Torques/External Force and Torque  EnableForceX=on  EnableForceY=on  EnableForceZ=off  EnableForce=off  ForceResolutionFrame=World  EnableTorqueX=off  EnableTorqueY=off  EnableTorqueZ=off  EnableTorque=off  TorqueResolutionFrame=AttachedFrame
  Friction Force Calculator : MATLAB Function  TreatAsAtomicUnit=on
  Friction Force Calculator1 : MATLAB Function  TreatAsAtomicUnit=on
  Friction Force Calculator2 : MATLAB Function  TreatAsAtomicUnit=on
  Friction Force Calculator3 : MATLAB Function  TreatAsAtomicUnit=on
  Friction Force Calculator4 : MATLAB Function  TreatAsAtomicUnit=on
  GP1 : sm_lib/Frames and Transforms/Rigid Transform  RotationMethod=None  FollAlignAxisA=+X  BaseAlignAxisA=+Y  FollAlignAxisB=+Y  BaseAlignAxisB=+Z  RotationStandardAxis=+Z  RotationAngle=0.0  RotationAngleUnits=deg  RotationArbitraryAxis=[0 0 1]  RotationSequenceAxes=FollowerAxes  RotationSequence=XYX  RotationSequenceAngles=[0 0 0]  RotationSequenceAnglesUnits=deg  RotationMatrix=[1 0 0; 0 1 0; 0 0 1]  Quaternion=[1 0 0 0]  TranslationMethod=None  TranslationCartesianOffset=[0 0 0]  TranslationCartesianOffsetUnits=m  TranslationStandardAxis=-X  TranslationStandardOffset=d/2  TranslationStandardOffsetUnits=m  TranslationROffset=0  TranslationROffsetUnits=m  TranslationThetaOffset=0  TranslationThetaOffsetUnits=deg  TranslationZOffset=0  TranslationZOffsetUnits=m
  GP{2..5} (4 alike) : sm_lib/Frames and Transforms/Rigid Transform  RotationMethod=None  FollAlignAxisA=+X  BaseAlignAxisA=+Y  FollAlignAxisB=+Y  BaseAlignAxisB=+Z  RotationStandardAxis=+Z  RotationAngle=0.0  RotationAngleUnits=deg  RotationArbitraryAxis=[0 0 1]  RotationSequenceAxes=FollowerAxes  RotationSequence=XYX  RotationSequenceAngles=[0 0 0]  RotationSequenceAnglesUnits=deg  RotationMatrix=[1 0 0; 0 1 0; 0 0 1]  Quaternion=[1 0 0 0]  TranslationMethod=StandardAxis  TranslationCartesianOffset=[0 0 0]  TranslationCartesianOffsetUnits=m  TranslationStandardAxis=+X  TranslationStandardOffset=footLength/4  TranslationStandardOffsetUnits=m  TranslationROffset=0  TranslationROffsetUnits=m  TranslationThetaOffset=0  TranslationThetaOffsetUnits=deg  TranslationZOffset=0  TranslationZOffsetUnits=m
  Normal Force Calculator : MATLAB Function  TreatAsAtomicUnit=on
  Normal Force Calculator1 : MATLAB Function  TreatAsAtomicUnit=on
  Normal Force Calculator2 : MATLAB Function  TreatAsAtomicUnit=on
  Normal Force Calculator3 : MATLAB Function  TreatAsAtomicUnit=on
  Normal Force Calculator4 : MATLAB Function  TreatAsAtomicUnit=on
  PS-Simulink Converter{1..15} (15 alike) : nesl_utility/PS-Simulink Converter  PhysicalDomain=network_engine_domain  SubClassName=ps_output  LeftPortType=input  RightPortType=output  PseudoPeriodic=off  Frequencies=[]  VectorFormat=1-D array  Unit=inherit  AffineConversion=off
  R_GRF : Scope
  Scope1 : Scope  NumInputPorts=5
  Scope2 : Scope  NumInputPorts=5
  Scope3 : Scope  NumInputPorts=5
  Simulink-PS Converter{,1..9} (10 alike) : nesl_utility/Simulink-PS Converter  PhysicalDomain=network_engine_domain  SubClassName=ps_input  LeftPortType=input  RightPortType=output  PseudoPeriodic=off  Frequencies=[]  NoiseDistribution=none  NoiseParameters=[]  Unit=1  AffineConversion=off  FilteringAndDerivatives=provide  SimscapeFilterOrder=1  InputFilterTimeConstant=0.001  UdotUserProvided=0
  Sum : Sum  Inputs=+++++
  Transform Sensor{,1..4} (5 alike) : sm_lib/Frames and Transforms/Transform Sensor  MeasurementFrame=World  RotationSequence=XYX  SenseAngle=off  SenseAxis=off  SenseQ=off  SenseR=off  SenseRotationSequence=off  SenseOmegaX=off  SenseOmegaY=off  SenseOmegaZ=off  SenseOmega=off  SenseQDot=off  SenseRDot=off  SenseRotationSequenceDot=off  SenseAlphaX=off  SenseAlphaY=off  SenseAlphaZ=off  SenseAlpha=off  SenseQDDot=off  SenseRDDot=off  SenseX=off  SenseY=on  SenseZ=off  SenseXYZ=off  SenseRad=off  SenseAzim=off  SenseDist=off  SenseInc=off  SenseXDot=on  SenseYDot=on  SenseZDot=off  SenseXYZDot=off  SenseRadDot=off  SenseAzimDot=off  SenseDistDot=off  SenseIncDot=off  SenseXDDot=off  SenseYDDot=off  SenseZDDot=off  SenseXYZDDot=off  SenseRadDDot=off  SenseAzimDDot=off  SenseDistDDot=off  SenseIncDDot=off
  World Frame : sm_lib/Frames and Transforms/World Frame
  Conn1 : PMIOPort  Side=Left
  wires:
  PS-Simulink Converter2/1 -> Scope1/1, Normal Force Calculator/3(u)
  Normal Force Calculator4/1(y) -> Sum/5, Scope2/5, Friction Force Calculator4/2(F_N), Simulink-PS Converter4/1
  Friction Force Calculator3/1(y) -> Scope3/4, Simulink-PS Converter8/1
  Normal Force Calculator/1(y) -> Sum/1, Scope2/1, Friction Force Calculator/2(F_N), Simulink-PS Converter/1
  PS-Simulink Converter9/1 -> Normal Force Calculator4/3(u), Scope1/5
  Friction Force Calculator4/1(y) -> Scope3/5, Simulink-PS Converter9/1
  PS-Simulink Converter5/1 -> Normal Force Calculator2/3(u), Scope1/3
  PS-Simulink Converter15/1 -> Friction Force Calculator4/1(u)
  PS-Simulink Converter10/1 -> Normal Force Calculator4/4(udot)
  PS-Simulink Converter8/1 -> Normal Force Calculator3/4(udot)
  PS-Simulink Converter12/1 -> Friction Force Calculator1/1(u)
  Normal Force Calculator1/1(y) -> Sum/2, Scope2/2, Friction Force Calculator1/2(F_N), Simulink-PS Converter1/1
  PS-Simulink Converter13/1 -> Friction Force Calculator2/1(u)
  PS-Simulink Converter3/1 -> Normal Force Calculator1/3(u), Scope1/2
  PS-Simulink Converter4/1 -> Normal Force Calculator1/4(udot)
  Friction Force Calculator2/1(y) -> Scope3/3, Simulink-PS Converter7/1
  PS-Simulink Converter1/1 -> Normal Force Calculator/4(udot)
  Friction Force Calculator/1(y) -> Scope3/1, Simulink-PS Converter5/1
  Normal Force Calculator3/1(y) -> Scope2/4, Sum/4, Friction Force Calculator3/2(F_N), Simulink-PS Converter3/1
  PS-Simulink Converter7/1 -> Normal Force Calculator3/3(u), Scope1/4
  Constant1/1 -> Normal Force Calculator4/2(c_max), Normal Force Calculator3/2(c_max), Normal Force Calculator2/2(c_max), Normal Force Calculator1/2(c_max), Normal Force Calculator/2(c_max)
  PS-Simulink Converter6/1 -> Normal Force Calculator2/4(udot)
  Normal Force Calculator2/1(y) -> Sum/3, Scope2/3, Friction Force Calculator2/2(F_N), Simulink-PS Converter2/1
  Friction Force Calculator1/1(y) -> Scope3/2, Simulink-PS Converter6/1
  Sum/1 -> R_GRF/1
  Constant/1 -> Normal Force Calculator3/1(k), Normal Force Calculator4/1(k), Normal Force Calculator2/1(k), Normal Force Calculator1/1(k), Normal Force Calculator/1(k)
  PS-Simulink Converter14/1 -> Friction Force Calculator3/1(u)
  PS-Simulink Converter11/1 -> Friction Force Calculator/1(u)
  connections:
  Simulink-PS Converter5/RConn1 -- External Force and Torque/LConn1
  External Force and Torque2/LConn2 -- Simulink-PS Converter2/RConn1
  GP3/RConn1 -- External Force and Torque2/RConn1 -- Transform Sensor2/RConn1 -- GP4/LConn1
  GP2/LConn1 -- External Force and Torque/RConn1 -- Transform Sensor/RConn1 -- GP1/RConn1
  Transform Sensor2/RConn4 -- PS-Simulink Converter6/LConn1
  World Frame/RConn1 -- Transform Sensor4/LConn1 -- Transform Sensor3/LConn1 -- Transform Sensor2/LConn1 -- Transform Sensor1/LConn1 -- Transform Sensor/LConn1
  Transform Sensor3/RConn4 -- PS-Simulink Converter8/LConn1
  External Force and Torque1/LConn1 -- Simulink-PS Converter6/RConn1
  Transform Sensor3/RConn3 -- PS-Simulink Converter14/LConn1
  Transform Sensor4/RConn1 -- External Force and Torque4/RConn1 -- GP5/RConn1
  External Force and Torque3/LConn2 -- Simulink-PS Converter3/RConn1
  GP4/RConn1 -- External Force and Torque3/RConn1 -- Transform Sensor3/RConn1 -- GP5/LConn1
  Transform Sensor/RConn2 -- PS-Simulink Converter2/LConn1
  Transform Sensor2/RConn3 -- PS-Simulink Converter13/LConn1
  GP3/LConn1 -- External Force and Torque1/RConn1 -- Transform Sensor1/RConn1 -- GP2/RConn1
  Simulink-PS Converter7/RConn1 -- External Force and Torque2/LConn1
  Simulink-PS Converter8/RConn1 -- External Force and Torque3/LConn1
  PS-Simulink Converter3/LConn1 -- Transform Sensor1/RConn2
  Simulink-PS Converter1/RConn1 -- External Force and Torque1/LConn2
  Transform Sensor/RConn4 -- PS-Simulink Converter1/LConn1
  Transform Sensor4/RConn4 -- PS-Simulink Converter10/LConn1
  Transform Sensor4/RConn2 -- PS-Simulink Converter9/LConn1
  Transform Sensor/RConn3 -- PS-Simulink Converter11/LConn1
  Transform Sensor1/RConn4 -- PS-Simulink Converter4/LConn1
  Simulink-PS Converter/RConn1 -- External Force and Torque/LConn2
  Transform Sensor3/RConn2 -- PS-Simulink Converter7/LConn1
  Transform Sensor2/RConn2 -- PS-Simulink Converter5/LConn1
  Simulink-PS Converter9/RConn1 -- External Force and Torque4/LConn1
  Transform Sensor1/RConn3 -- PS-Simulink Converter12/LConn1
  Transform Sensor4/RConn3 -- PS-Simulink Converter15/LConn1
  External Force and Torque4/LConn2 -- Simulink-PS Converter4/RConn1
  GP1/LConn1 -- Conn1/RConn1

== system ABMS_FK_Optimization/R. Leg Inputs/Subsystem ==
  In1 : Inport
  Demux1 : Demux  Outputs=2
  From Workspace1 : FromWorkspace  VariableName=[t1.',theta_knee_R ]  SampleTime=dt
  From Workspace5 : FromWorkspace  VariableName=[t1.',omega_knee_R]  SampleTime=dt
  Gain2 : Gain  Gain=kKnee
  Gain3 : Gain  Gain=cKnee
  Subtract2 : Sum  Inputs=+-
  Subtract3 : Sum  Inputs=+-
  Sum1 : Sum  Inputs=|++
  Out1 : Outport
  wires:
  Subtract2/1 -> Gain2/1
  Gain3/1 -> Sum1/2
  Gain2/1 -> Sum1/1
  Demux1/1 -> Subtract2/2
  Demux1/2 -> Subtract3/2
  Subtract3/1 -> Gain3/1
  From Workspace5/1 -> Subtract3/1
  From Workspace1/1 -> Subtract2/1
  In1/1 -> Demux1/1
  Sum1/1 -> Out1/1

== system ABMS_FK_Optimization/R. Leg Inputs/Subsystem1 ==
  In1 : Inport
  Demux : Demux  Outputs=2
  From Workspace7 : FromWorkspace  VariableName=[t1.',theta_ankle_R]  SampleTime=dt
  From Workspace8 : FromWorkspace  VariableName=[t1.',omega_ankle_R]  SampleTime=dt
  Gain : Gain  Gain=kAnkle
  Gain1 : Gain  Gain=cAnkle
  Subtract : Sum  Inputs=+-
  Subtract1 : Sum  Inputs=+-
  Sum : Sum  Inputs=|++
  Out1 : Outport
  wires:
  From Workspace7/1 -> Subtract/1
  Subtract/1 -> Gain/1
  From Workspace8/1 -> Subtract1/1
  Demux/1 -> Subtract/2
  Demux/2 -> Subtract1/2
  Gain1/1 -> Sum/2
  Gain/1 -> Sum/1
  Subtract1/1 -> Gain1/1
  In1/1 -> Demux/1
  Sum/1 -> Out1/1

== system ABMS_FK_Optimization/R. Leg Inputs/Subsystem2 ==
  1 : Inport
  Demux : Demux  Outputs=2
  From Workspace : FromWorkspace  VariableName=[t1.',theta_hip_R]  SampleTime=dt
  From Workspace3 : FromWorkspace  VariableName=[t1.',omega_hip_R]  SampleTime=dt
  Gain : Gain  Gain=kHip
  Gain1 : Gain  Gain=cHip
  Subtract : Sum  Inputs=+-
  Subtract1 : Sum  Inputs=+-
  Sum : Sum  Inputs=|++
  Out1 : Outport
  wires:
  From Workspace/1 -> Subtract/1
  Subtract/1 -> Gain/1
  From Workspace3/1 -> Subtract1/1
  Demux/1 -> Subtract/2
  Demux/2 -> Subtract1/2
  Gain1/1 -> Sum/2
  Gain/1 -> Sum/1
  Subtract1/1 -> Gain1/1
  1/1 -> Demux/1
  Sum/1 -> Out1/1

== matlab function ABMS_FK_Optimization/R. Leg/GRF/Normal Force Calculator1 ==
  data: k input; c_max input; u input; y output; udot input
function y = fcn(k, c_max, u, udot)

%k = 1.5e4;
%c_max = 1500;
h = 0.01;

d = abs(u);
ddot = abs(udot);

    if u <= 0
        F_k = k*d;
        if d < h
            F_c = c_max*abs(3*(d/h)^2-2*(d/h)^3)*ddot;
        else
            F_c = c_max*ddot;
        end 
    else
        F_k = 0;
        F_c = 0;
    end

y = F_k + F_c;

== matlab function ABMS_FK_Optimization/L. Leg/GRF/Friction Force Calculator ==
  data: u input; y output; F_N input
function y = fcn(u, F_N)

    mu_s = 0.8;
    mu_d = 0.2;
    
    if sign(u) == 0
        S = 1;
    else
        S = sign(u);
    end
    
    if u < 0.05
        mu = mu_s;
    else
        mu = mu_d;
    end
y = -mu*S*F_N;

== matlab function ABMS_FK_Optimization/L. Leg/GRF/Friction Force Calculator1 ==
  data: u input; y output; F_N input
function y = fcn(u, F_N)

    mu_s = 0.8;
    mu_d = 0.2;
    
    if sign(u) == 0
        S = 1;
    else
        S = sign(u);
    end
    
    if u < 0.05
        mu = mu_s;
    else
        mu = mu_d;
    end
y = -mu*S*F_N;

== matlab function ABMS_FK_Optimization/L. Leg/GRF/Friction Force Calculator2 ==
  data: u input; y output; F_N input
function y = fcn(u, F_N)

    mu_s = 0.8;
    mu_d = 0.2;
    
    if sign(u) == 0
        S = 1;
    else
        S = sign(u);
    end
    
    if u < 0.05
        mu = mu_s;
    else
        mu = mu_d;
    end
y = -mu*S*F_N;

== matlab function ABMS_FK_Optimization/L. Leg/GRF/Friction Force Calculator3 ==
  data: u input; y output; F_N input
function y = fcn(u, F_N)

    mu_s = 0.8;
    mu_d = 0.2;
    
    if sign(u) == 0
        S = 1;
    else
        S = sign(u);
    end
    
    if u < 0.05
        mu = mu_s;
    else
        mu = mu_d;
    end
y = -mu*S*F_N;

== matlab function ABMS_FK_Optimization/L. Leg/GRF/Friction Force Calculator4 ==
  data: u input; y output; F_N input
function y = fcn(u, F_N)

    mu_s = 0.8;
    mu_d = 0.2;
    
    if sign(u) == 0
        S = 1;
    else
        S = sign(u);
    end
    
    if u < 0.05
        mu = mu_s;
    else
        mu = mu_d;
    end
y = -mu*S*F_N;

== matlab function ABMS_FK_Optimization/L. Leg/GRF/Normal Force Calculator ==
  data: k input; c_max input; u input; y output; udot input
function y = fcn(k, c_max, u, udot)

%k = 1.5e4;
%c_max = 1500;
h = 0.01;

d = abs(u);
ddot = abs(udot);

    if u <= 0
        F_k = k*d;
        if d < h
            F_c = c_max*abs(3*(d/h)^2-2*(d/h)^3)*ddot;
        else
            F_c = c_max*ddot;
        end 
    else
        F_k = 0;
        F_c = 0;
    end

y = F_k + F_c;

== matlab function ABMS_FK_Optimization/L. Leg/GRF/Normal Force Calculator1 ==
  data: k input; c_max input; u input; y output; udot input
function y = fcn(k, c_max, u, udot)

%k = 1.5e4;
%c_max = 1500;
h = 0.01;

d = abs(u);
ddot = abs(udot);

    if u <= 0
        F_k = k*d;
        if d < h
            F_c = c_max*abs(3*(d/h)^2-2*(d/h)^3)*ddot;
        else
            F_c = c_max*ddot;
        end 
    else
        F_k = 0;
        F_c = 0;
    end

y = F_k + F_c;

== matlab function ABMS_FK_Optimization/L. Leg/GRF/Normal Force Calculator2 ==
  data: k input; c_max input; u input; y output; udot input
function y = fcn(k, c_max, u, udot)

%k = 1.5e4;
%c_max = 1500;
h = 0.01;

d = abs(u);
ddot = abs(udot);

    if u <= 0
        F_k = k*d;
        if d < h
            F_c = c_max*abs(3*(d/h)^2-2*(d/h)^3)*ddot;
        else
            F_c = c_max*ddot;
        end 
    else
        F_k = 0;
        F_c = 0;
    end

y = F_k + F_c;

== matlab function ABMS_FK_Optimization/L. Leg/GRF/Normal Force Calculator3 ==
  data: k input; c_max input; u input; y output; udot input
function y = fcn(k, c_max, u, udot)

%k = 1.5e4;
%c_max = 1500;
h = 0.01;

d = abs(u);
ddot = abs(udot);

    if u <= 0
        F_k = k*d;
        if d < h
            F_c = c_max*abs(3*(d/h)^2-2*(d/h)^3)*ddot;
        else
            F_c = c_max*ddot;
        end 
    else
        F_k = 0;
        F_c = 0;
    end

y = F_k + F_c;

== matlab function ABMS_FK_Optimization/L. Leg/GRF/Normal Force Calculator4 ==
  data: k input; c_max input; u input; y output; udot input
function y = fcn(k, c_max, u, udot)

%k = 1.5e4;
%c_max = 1500;
h = 0.01;

d = abs(u);
ddot = abs(udot);

    if u <= 0
        F_k = k*d;
        if d < h
            F_c = c_max*abs(3*(d/h)^2-2*(d/h)^3)*ddot;
        else
            F_c = c_max*ddot;
        end 
    else
        F_k = 0;
        F_c = 0;
    end

y = F_k + F_c;

== matlab function ABMS_FK_Optimization/R. Leg/GRF/Normal Force Calculator ==
  data: k input; c_max input; u input; y output; udot input
function y = fcn(k, c_max, u, udot)

%k = 1.5e4;
%c_max = 1500;
h = 0.01;

d = abs(u);
ddot = abs(udot);

    if u <= 0
        F_k = k*d;
        if d < h
            F_c = c_max*abs(3*(d/h)^2-2*(d/h)^3)*ddot;
        else
            F_c = c_max*ddot;
        end 
    else
        F_k = 0;
        F_c = 0;
    end

y = F_k + F_c;
